simulink subsystem "INA219_Current_Sensor"  (R2022b)
settings: Solver=VariableStepAuto  StartTime=0.0  StopTime=10.0  RelTol=1e-3
undefined symbols (not defined in the file or in its folder): cf
libraries: simulink x2
settings Model: Creator=gotta  LastModifiedBy=gotta

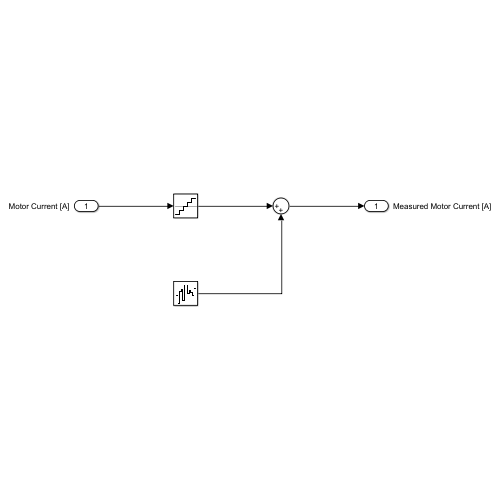
[thumbnail: Simulink's stored preview of the top-level diagram]
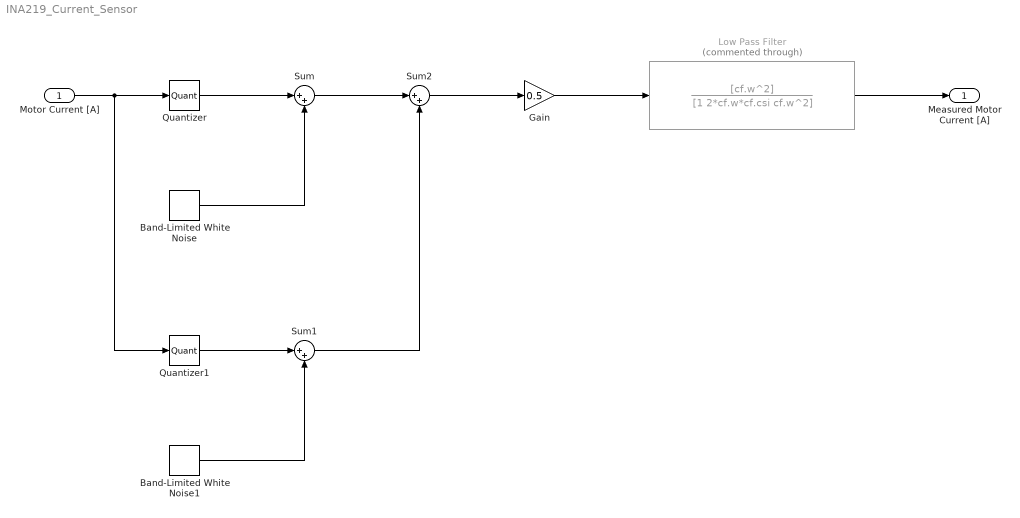
== system INA219_Current_Sensor ==
  Motor Current [A] : Inport
  Band-Limited White Noise : simulink/Sources/Band-Limited White Noise  Cov=[1e-8]  Ts=1e-3  seed=[23341]
  Band-Limited White Noise1 : simulink/Sources/Band-Limited White Noise  Cov=[1e-8]  Ts=1e-3  seed=[24560]
  Gain : Gain  Gain=0.5
  Low Pass Filter : TransferFcn  Commented=through  Numerator=[cf.w^2]  Denominator=[1 2*cf.w*cf.csi cf.w^2]
  Quantizer : Quantizer  QuantizationInterval=INA219.current_LSB
  Quantizer1 : Quantizer  QuantizationInterval=INA219.current_LSB
  Sum : Sum  Inputs=|++
  Sum1 : Sum  Inputs=|++
  Sum2 : Sum  Inputs=|++
  Measured Motor Current [A] : Outport
  wires:
  Quantizer/1 -> Sum/1
  Band-Limited White Noise/1 -> Sum/2
  Sum1/1 -> Sum2/2
  Band-Limited White Noise1/1 -> Sum1/2
  Quantizer1/1 -> Sum1/1
  Motor Current [A]/1 -> Quantizer/1, Quantizer1/1
  Sum/1 -> Sum2/1
  Sum2/1 -> Gain/1
  Gain/1 -> Low Pass Filter/1
  Low Pass Filter/1 -> Measured Motor Current [A]/1
